simulink subsystem "RoboRio_Controls_sub"  (R2023b)
settings: Solver=VariableStepAuto  StartTime=0.0  StopTime=10.0  RelTol=1e-3
libraries: Autonomous_lib x1, simulink_extras x1, Disabled_lib x1, Teleop_lib x1, Test_lib x1
settings Model: Creator=USER  LastModifiedBy=FIRSTMentor

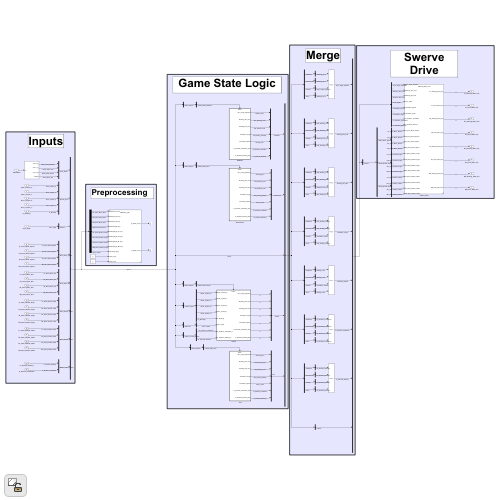
[thumbnail: Simulink's stored preview of the top-level diagram]
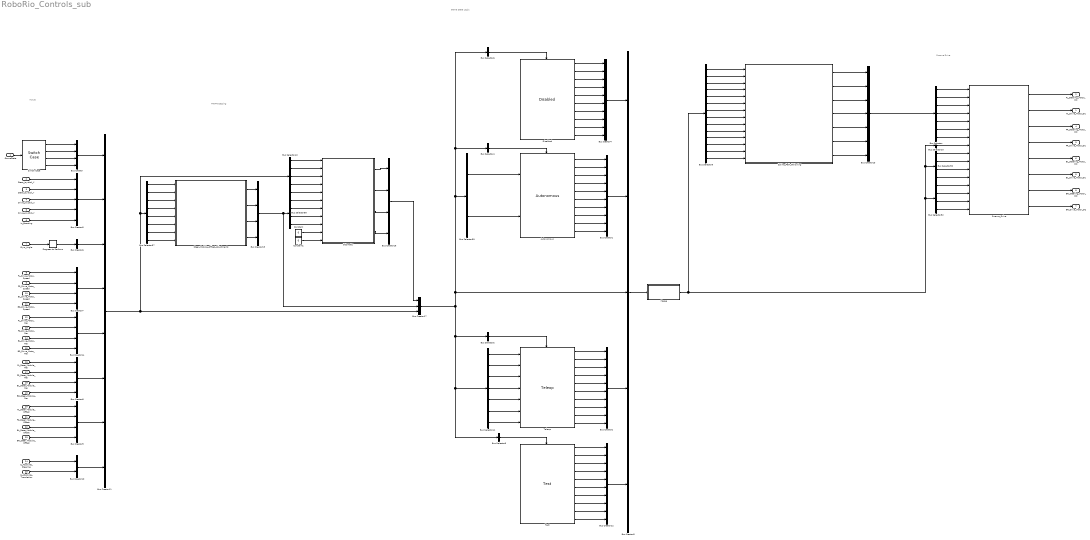
== system RoboRio_Controls_sub ==
  note: Game State Logic
  note: Swerve Drive
  note: Inputs
  note: Pre-Processing
  GameState : Inport
  Steer_Joystick_X : Inport  Port=2
  Steer_Joystick_Y : Inport  Port=3
  Drive_Joystick_X : Inport  Port=4
  Drive_Joystick_Y : Inport  Port=5
  Is_Boosting : Inport  Port=6
  Gyro_Angle : Inport  Port=7
  FL_Drive_Motor_Speed : Inport  Port=8
  FR_Drive_Motor_Speed : Inport  Port=9
  BL_Drive_Motor_Speed : Inport  Port=10
  BR_Drive_Motor_Speed : Inport  Port=11
  FL_Drive_Motor_Rev : Inport  Port=12
  FR_Drive_Motor_Rev : Inport  Port=13
  BL_Drive_Motor_Rev : Inport  Port=14
  BR_Drive_Motor_Rev : Inport  Port=15
  FL_Steer_Module_Rev : Inport  Port=16
  FR_Steer_Module_Rev : Inport  Port=17
  BL_Steer_Module_Rev : Inport  Port=18
  BR_Steer_Module_Rev : Inport  Port=19
  FL_Steer_Module_Offset : Inport  Port=20
  FR_Steer_Module_Offset : Inport  Port=21
  BL_Steer_Module_Offset : Inport  Port=22
  BR_Steer_Module_Offset : Inport  Port=23
  Is_Absolute_Steering : Inport  Port=24
  Is_Absolute_Translation : Inport  Port=25
  Autonomous : Autonomous_lib/Autonomous  SystemSampleTime=-1  VariantActivationTime=update diagram  AllowFlexibleInterface=on  Latency=0  AutoFrameSizeCalculation=off
  Bus Creator{,7..9,14..16} (7 alike) : BusCreator  Inputs=4
  Bus Creator{1..2,4,12} (4 alike) : BusCreator  Inputs=10
  Bus Creator10 : BusCreator  Inputs=2
  Bus Creator11 : BusCreator  Inputs=8
  Bus Creator13 : BusCreator  Inputs=7
  Bus Creator17 : BusCreator  Inputs=3
  Bus Creator3 : BusCreator  Inputs=5
  Bus Creator5 : BusCreator  Inputs=5
  Bus Creator6 : BusCreator  Inputs=1
  Bus Selector : BusSelector  OutputSignals=Steering_Abs_Cmd,Steering_Rel_Cmd,Translation_Speed,Translation_Angle,Is_Absolute_Translation,Is_Absolute_Steering,Gyro_Angle_Adjustment
  Bus Selector10 : BusSelector  OutputSignals=PreProcessing.Inputs.Sensors.Gyro_Angle
  Bus Selector2 : BusSelector  OutputSignals=Inputs.Game_States.Game_State_Teleop
  Bus Selector4 : BusSelector  OutputSignals=Inputs.Game_States.Game_State_Auto
  Bus Selector40 : BusSelector  OutputSignals=Sensors.Gyro_Angle,Drive_Motor_Revs.FL_Drive_Motor_Rev,Drive_Motor_Revs.FR_Drive_Motor_Rev,Drive_Motor_Revs.BL_Drive_Motor_Rev,Drive_Motor_Revs.BR_Drive_Motor_Rev
  Bus Selector41 : BusSelector  OutputSignals=Inputs.Human_Inputs.Steer_Joystick_X,Inputs.Human_Inputs.Steer_Joystick_Y,Inputs.Human_Inputs.Drive_Joystick_X,Inputs.Human_Inputs.Drive_Joystick_Y,Inputs.Human_Inputs.Is_Boosting,Inputs.Motion_Control_Modes.Is_Absolute_Translation,Inputs.Motion_Control_Modes.Is_Absolute_Steering
  Bus Selector50 : BusSelector  OutputSignals=PreProcessing.Inputs.Drive_Motor_Speeds.FL_Drive_Motor_Speed,PreProcessing.Inputs.Drive_Motor_Speeds.FR_Drive_Motor_Speed,PreProcessing.Inputs.Drive_Motor_Speeds.BL_Drive_Motor_Speed,PreProcessing.Inputs.Drive_Motor_Speeds.BR_Drive_Motor_Speed
  Bus Selector52 : BusSelector  OutputSignals=PreProcessing.Steer_Module_Angles.FL_Steer_Module_Angle,PreProcessing.Steer_Module_Angles.FR_Steer_Module_Angle,PreProcessing.Steer_Module_Angles.BL_Steer_Module_Angle,PreProcessing.Steer_Module_Angles.BR_Steer_Module_Angle
  Bus Selector57 : BusSelector  OutputSignals=Steer_Module_Revs.FL_Steer_Module_Rev,Steer_Module_Offsets.FL_Steer_Module_Offset,Steer_Module_Revs.FR_Steer_Module_Rev,Steer_Module_Offsets.FR_Steer_Module_Offset,Steer_Module_Revs.BL_Steer_Module_Rev,Steer_Module_Offsets.BL_Steer_Module_Offset,Steer_Module_Revs.BR_Steer_Module_Rev,Steer_Module_Offsets.BR_Steer_Module_Offset
  Bus Selector58 : BusSelector  OutputSignals=FL_Steer_Module_Angle,FR_Steer_Module_Angle,BL_Steer_Module_Angle,BR_Steer_Module_Angle
  Bus Selector59 : BusSelector  OutputSignals=Odometry.Odom_Position_X_global,Odometry.Odom_Position_Y_global
  Bus Selector6 : BusSelector  OutputSignals=Inputs.Game_States.Game_State_Disabled
  Bus Selector8 : BusSelector  OutputSignals=Inputs.Game_States.Game_State_Test
  Bus Selector9 : BusSelector  OutputSignals=Spline_Enable,Spline_Ref_Poses,Spline_Num_Poses,PreProcessing.Odometry.Odom_Position_X_global,PreProcessing.Odometry.Odom_Position_Y_global,PreProcessing.Odometry.Odom_Velocity_X_global,PreProcessing.Odometry.Odom_Velocity_Y_global,Steering_Abs_Cmd,Steering_Rel_Cmd,Translation_Speed,Translation_Angle,Is_Absolute_Translation,Is_Absolute_Steering,Gyro_Angle_Adjustment
  Constant : Constant  Value=0
  Constant1 : Constant  Value=0
  Degrees to Radians : simulink_extras/Transformations/Degrees to Radians
  Disabled : Disabled_lib/Disabled  SystemSampleTime=-1  VariantActivationTime=update diagram  AllowFlexibleInterface=on  Latency=0  AutoFrameSizeCalculation=off
  Merge : Subsystem
  Odometry : Subsystem  ReferencedSubsystem=Odometry_sub
  Spline_Path_Following : Subsystem  ReferencedSubsystem=Spline_Path_Following_sub
  Steer_Module_Offset_Adjustments : Subsystem  ReferencedSubsystem=Steer_Module_Offset_Adjustments_sub
  Swerve_Drive : Subsystem  ReferencedSubsystem=Swerve_Drive_sub
  Switch Case : SwitchCase  CaseConditions={0,1,2}
  Teleop : Teleop_lib/Teleop  SystemSampleTime=-1  VariantActivationTime=update diagram  AllowFlexibleInterface=on  Latency=0  AutoFrameSizeCalculation=off
  Test : Test_lib/Test  SystemSampleTime=-1  VariantActivationTime=update diagram  AllowFlexibleInterface=on  Latency=0  AutoFrameSizeCalculation=off
  FL_Drive_Motor_DC : Outport
  FL_Steering_Motor_DC : Outport  Port=2
  FR_Drive_Motor_DC : Outport  Port=3
  FR_Steering_Motor_DC : Outport  Port=4
  BL_Drive_Motor_DC : Outport  Port=5
  BL_Steering_Motor_DC : Outport  Port=6
  BR_Drive_Motor_DC : Outport  Port=7
  BR_Steering_Motor_DC : Outport  Port=8
  wires:
  Teleop/1 -> Bus Creator2/1
  Teleop/2 -> Bus Creator2/2
  Teleop/3 -> Bus Creator2/3
  Teleop/4 -> Bus Creator2/4
  Teleop/5 -> Bus Creator2/5
  Bus Creator4/1 -> Bus Creator3/1  "Disabled"
  Bus Creator1/1 -> Bus Creator3/2  "Autonomous"
  Bus Creator2/1 -> Bus Creator3/4  "Teleop"
  Switch Case/1 -> Bus Creator/1  "Game_State_Disabled"
  Switch Case/2 -> Bus Creator/2  "Game_State_Auto"
  Switch Case/3 -> Bus Creator/3  "Game_State_Teleop"
  GameState/1 -> Switch Case/1
  Bus Creator12/1 -> Bus Creator3/5  "Test"
  Switch Case/4 -> Bus Creator/4  "Game_State_Test"
  Steer_Joystick_Y/1 -> Bus Creator5/2  "Steer_Joystick_Y"
  Steer_Joystick_X/1 -> Bus Creator5/1  "Steer_Joystick_X"
  Drive_Joystick_X/1 -> Bus Creator5/3  "Drive_Joystick_X"
  Drive_Joystick_Y/1 -> Bus Creator5/4  "Drive_Joystick_Y"
  Gyro_Angle/1 -> Degrees to Radians/1
  Bus Creator5/1 -> Bus Creator11/2  "Human_Inputs"
  Bus Creator6/1 -> Bus Creator11/3  "Sensors"
  FL_Drive_Motor_Speed/1 -> Bus Creator7/1  "FL_Drive_Motor_Speed"
  FR_Drive_Motor_Speed/1 -> Bus Creator7/2  "FR_Drive_Motor_Speed"
  BL_Drive_Motor_Speed/1 -> Bus Creator7/3  "BL_Drive_Motor_Speed"
  BR_Drive_Motor_Speed/1 -> Bus Creator7/4  "BR_Drive_Motor_Speed"
  FL_Steer_Module_Rev/1 -> Bus Creator8/1  "FL_Steer_Module_Rev"
  BL_Steer_Module_Rev/1 -> Bus Creator8/3  "BL_Steer_Module_Rev"
  BR_Steer_Module_Rev/1 -> Bus Creator8/4  "BR_Steer_Module_Rev"
  FR_Steer_Module_Rev/1 -> Bus Creator8/2  "FR_Steer_Module_Rev"
  Bus Creator7/1 -> Bus Creator11/4  "Drive_Motor_Speeds"
  Bus Creator8/1 -> Bus Creator11/6  "Steer_Module_Revs"
  FL_Steer_Module_Offset/1 -> Bus Creator9/1  "FL_Steer_Module_Offset"
  FR_Steer_Module_Offset/1 -> Bus Creator9/2  "FR_Steer_Module_Offset"
  BL_Steer_Module_Offset/1 -> Bus Creator9/3  "BL_Steer_Module_Offset"
  BR_Steer_Module_Offset/1 -> Bus Creator9/4  "BR_Steer_Module_Offset"
  Bus Creator9/1 -> Bus Creator11/7  "Steer_Module_Offsets"
  Is_Absolute_Steering/1 -> Bus Creator10/1  "Is_Absolute_Steering"
  Is_Absolute_Translation/1 -> Bus Creator10/2  "Is_Absolute_Translation"
  Bus Creator10/1 -> Bus Creator11/8  "Motion_Control_Modes"
  Bus Selector41/1 -> Teleop/1  "<Steer_Joystick_X>"
  Bus Selector41/2 -> Teleop/2  "<Steer_Joystick_Y>"
  Bus Selector41/3 -> Teleop/3  "<Drive_Joystick_X>"
  Bus Selector41/4 -> Teleop/4  "<Drive_Joystick_Y>"
  Teleop/6 -> Bus Creator2/6
  Teleop/7 -> Bus Creator2/7
  Autonomous/2 -> Bus Creator1/2
  Autonomous/4 -> Bus Creator1/4
  Autonomous/1 -> Bus Creator1/1
  Autonomous/5 -> Bus Creator1/5
  Autonomous/7 -> Bus Creator1/7
  Autonomous/3 -> Bus Creator1/3
  Autonomous/6 -> Bus Creator1/6
  Disabled/2 -> Bus Creator4/2
  Disabled/4 -> Bus Creator4/4
  Disabled/1 -> Bus Creator4/1
  Disabled/5 -> Bus Creator4/5
  Disabled/7 -> Bus Creator4/7
  Disabled/3 -> Bus Creator4/3
  Disabled/6 -> Bus Creator4/6
  Test/2 -> Bus Creator12/2
  Test/4 -> Bus Creator12/4
  Test/1 -> Bus Creator12/1
  Test/5 -> Bus Creator12/5
  Test/7 -> Bus Creator12/7
  Test/3 -> Bus Creator12/3
  Test/6 -> Bus Creator12/6
  Bus Creator/1 -> Bus Creator11/1  "Game_States"
  Bus Selector2/1 -> Teleop/Action  "<Game_State_Teleop>"
  Bus Selector4/1 -> Autonomous/Action  "<Game_State_Auto>"
  Bus Selector6/1 -> Disabled/Action  "<Game_State_Disabled>"
  Bus Selector8/1 -> Test/Action  "<Game_State_Test>"
  Bus Selector50/4 -> Swerve_Drive/12  "<BR_Drive_Motor_Speed>"
  Bus Selector50/3 -> Swerve_Drive/11  "<BL_Drive_Motor_Speed>"
  Bus Selector50/2 -> Swerve_Drive/10  "<FR_Drive_Motor_Speed>"
  Bus Selector50/1 -> Swerve_Drive/9  "<FL_Drive_Motor_Speed>"
  Swerve_Drive/1 -> FL_Steering_Motor_DC/1
  Swerve_Drive/2 -> FL_Drive_Motor_DC/1
  Swerve_Drive/3 -> FR_Steering_Motor_DC/1
  Swerve_Drive/4 -> FR_Drive_Motor_DC/1
  Swerve_Drive/5 -> BL_Steering_Motor_DC/1
  Swerve_Drive/6 -> BL_Drive_Motor_DC/1
  Swerve_Drive/7 -> BR_Steering_Motor_DC/1
  Swerve_Drive/8 -> BR_Drive_Motor_DC/1
  Is_Boosting/1 -> Bus Creator5/5  "Is_Boosting"
  Bus Selector41/5 -> Teleop/5  "<Is_Boosting>"
  Bus Creator14/1 -> Bus Creator11/5  "Drive_Motor_Revs"
  FL_Drive_Motor_Rev/1 -> Bus Creator14/1  "FL_Drive_Motor_Rev"
  FR_Drive_Motor_Rev/1 -> Bus Creator14/2  "FR_Drive_Motor_Rev"
  BL_Drive_Motor_Rev/1 -> Bus Creator14/3  "BL_Drive_Motor_Rev"
  BR_Drive_Motor_Rev/1 -> Bus Creator14/4  "BR_Drive_Motor_Rev"
  Bus Selector40/2 -> Odometry/2  "<FL_Drive_Motor_Rev>"
  Bus Selector40/3 -> Odometry/3  "<FR_Drive_Motor_Rev>"
  Bus Selector40/4 -> Odometry/4  "<BL_Drive_Motor_Rev>"
  Bus Selector40/5 -> Odometry/5  "<BR_Drive_Motor_Rev>"
  Bus Selector40/1 -> Odometry/1  "<Gyro_Angle>"
  Constant1/1 -> Odometry/11
  Constant/1 -> Odometry/10
  Bus Selector57/1 -> Steer_Module_Offset_Adjustments/1  "<FL_Steer_Module_Rev>"
  Bus Selector57/2 -> Steer_Module_Offset_Adjustments/2  "<FL_Steer_Module_Offset>"
  Bus Selector57/3 -> Steer_Module_Offset_Adjustments/3  "<FR_Steer_Module_Rev>"
  Bus Selector57/4 -> Steer_Module_Offset_Adjustments/4  "<FR_Steer_Module_Offset>"
  Bus Selector57/5 -> Steer_Module_Offset_Adjustments/5  "<BL_Steer_Module_Rev>"
  Bus Selector57/6 -> Steer_Module_Offset_Adjustments/6  "<BL_Steer_Module_Offset>"
  Bus Selector57/7 -> Steer_Module_Offset_Adjustments/7  "<BR_Steer_Module_Rev>"
  Bus Selector57/8 -> Steer_Module_Offset_Adjustments/8  "<BR_Steer_Module_Offset>"
  Steer_Module_Offset_Adjustments/2 -> Bus Creator15/2
  Steer_Module_Offset_Adjustments/1 -> Bus Creator15/1
  Steer_Module_Offset_Adjustments/3 -> Bus Creator15/3
  Steer_Module_Offset_Adjustments/4 -> Bus Creator15/4
  Bus Creator15/1 -> Bus Selector58/1, Bus Creator17/2  "Steer_Module_Angles"
  Bus Selector58/1 -> Odometry/6  "<FL_Steer_Module_Angle>"
  Bus Selector58/2 -> Odometry/7  "<FR_Steer_Module_Angle>"
  Bus Selector58/3 -> Odometry/8  "<BL_Steer_Module_Angle>"
  Bus Selector58/4 -> Odometry/9  "<BR_Steer_Module_Angle>"
  Odometry/1 -> Bus Creator16/1
  Odometry/2 -> Bus Creator16/2
  Bus Creator16/1 -> Bus Creator17/1  "Odometry"
  Bus Creator11/1 -> Bus Creator17/3, Bus Selector57/1, Bus Selector40/1  "Inputs"
  Bus Selector52/1 -> Swerve_Drive/13  "<FL_Steer_Module_Angle>"
  Bus Selector52/2 -> Swerve_Drive/14  "<FR_Steer_Module_Angle>"
  Bus Selector52/3 -> Swerve_Drive/15  "<BL_Steer_Module_Angle>"
  Bus Selector52/4 -> Swerve_Drive/16  "<BR_Steer_Module_Angle>"
  Degrees to Radians/1 -> Bus Creator6/1  "Gyro_Angle"
  Bus Creator17/1 -> Bus Selector8/1, Bus Selector41/1, Bus Selector2/1, Bus Creator3/3, Bus Selector59/1, Bus Selector4/1, Bus Selector6/1  "PreProcessing"
  Disabled/8 -> Bus Creator4/8
  Disabled/9 -> Bus Creator4/9
  Disabled/10 -> Bus Creator4/10
  Autonomous/8 -> Bus Creator1/8
  Autonomous/9 -> Bus Creator1/9
  Autonomous/10 -> Bus Creator1/10
  Teleop/8 -> Bus Creator2/8
  Teleop/9 -> Bus Creator2/9
  Teleop/10 -> Bus Creator2/10
  Test/8 -> Bus Creator12/8
  Test/9 -> Bus Creator12/9
  Test/10 -> Bus Creator12/10
  Merge/1(Bus_Out) -> Bus Selector52/1, Bus Selector50/1, Bus Selector10/1, Bus Selector9/1
  Bus Creator3/1 -> Merge/1(Bus_In)
  Odometry/3 -> Bus Creator16/3
  Odometry/4 -> Bus Creator16/4
  Bus Selector10/1 -> Swerve_Drive/8  "<Gyro_Angle>"
  Bus Selector59/1 -> Autonomous/1  "<Odom_Position_X_global>"
  Bus Selector59/2 -> Autonomous/2  "<Odom_Position_Y_global>"
  Bus Selector41/7 -> Teleop/7  "<Is_Absolute_Steering>"
  Bus Selector41/6 -> Teleop/6  "<Is_Absolute_Translation>"
  Bus Selector9/1 -> Spline_Path_Following/1  "<Spline_Enable>"
  Bus Selector9/2 -> Spline_Path_Following/2  "<Spline_Ref_Poses>"
  Bus Selector9/3 -> Spline_Path_Following/3  "<Spline_Num_Poses>"
  Bus Selector9/4 -> Spline_Path_Following/4  "<Odom_Position_X_global>"
  Bus Selector9/5 -> Spline_Path_Following/5  "<Odom_Position_Y_global>"
  Bus Selector9/6 -> Spline_Path_Following/6  "<Odom_Velocity_X_global>"
  Bus Selector9/7 -> Spline_Path_Following/7  "<Odom_Velocity_Y_global>"
  Bus Selector9/8 -> Spline_Path_Following/8  "<Steering_Abs_Cmd>"
  Bus Selector9/9 -> Spline_Path_Following/9  "<Steering_Rel_Cmd>"
  Bus Selector9/10 -> Spline_Path_Following/10  "<Translation_Speed>"
  Bus Selector9/11 -> Spline_Path_Following/11  "<Translation_Angle>"
  Bus Selector9/12 -> Spline_Path_Following/12  "<Is_Absolute_Translation>"
  Bus Selector9/13 -> Spline_Path_Following/13  "<Is_Absolute_Steering>"
  Bus Selector9/14 -> Spline_Path_Following/14  "<Gyro_Angle_Adjustment>"
  Spline_Path_Following/1 -> Bus Creator13/1
  Spline_Path_Following/2 -> Bus Creator13/2
  Spline_Path_Following/3 -> Bus Creator13/3
  Spline_Path_Following/4 -> Bus Creator13/4
  Spline_Path_Following/5 -> Bus Creator13/5
  Spline_Path_Following/6 -> Bus Creator13/6
  Spline_Path_Following/7 -> Bus Creator13/7
  Bus Creator13/1 -> Bus Selector/1
  Bus Selector/5 -> Swerve_Drive/5  "<Is_Absolute_Translation>"
  Bus Selector/4 -> Swerve_Drive/4  "<Translation_Angle>"
  Bus Selector/6 -> Swerve_Drive/6  "<Is_Absolute_Steering>"
  Bus Selector/3 -> Swerve_Drive/3  "<Translation_Speed>"
  Bus Selector/7 -> Swerve_Drive/7  "<Gyro_Angle_Adjustment>"
  Bus Selector/2 -> Swerve_Drive/2  "<Steering_Rel_Cmd>"
  Bus Selector/1 -> Swerve_Drive/1  "<Steering_Abs_Cmd>"

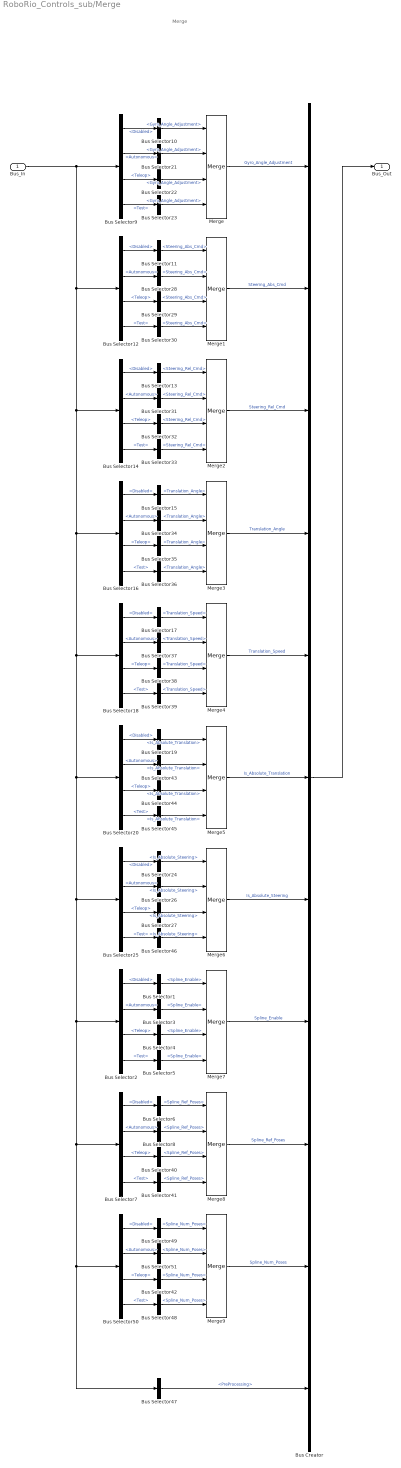
== system RoboRio_Controls_sub/Merge ==
  note: Merge
  Bus_In : Inport
  Bus Creator : BusCreator  Inputs=11
  Bus Selector{1,3..5} (4 alike) : BusSelector  OutputSignals=Spline_Enable
  Bus Selector{10,21..23} (4 alike) : BusSelector  OutputSignals=Gyro_Angle_Adjustment
  Bus Selector{11,28..30} (4 alike) : BusSelector  OutputSignals=Steering_Abs_Cmd
  Bus Selector{2,7,9,12,14,16,18,20,25,50} (10 alike) : BusSelector  OutputSignals=Disabled,Autonomous,Teleop,Test
  Bus Selector{13,31..33} (4 alike) : BusSelector  OutputSignals=Steering_Rel_Cmd
  Bus Selector{15,34..36} (4 alike) : BusSelector  OutputSignals=Translation_Angle
  Bus Selector{17,37..39} (4 alike) : BusSelector  OutputSignals=Translation_Speed
  Bus Selector{19,43..45} (4 alike) : BusSelector  OutputSignals=Is_Absolute_Translation
  Bus Selector{24,26..27,46} (4 alike) : BusSelector  OutputSignals=Is_Absolute_Steering
  Bus Selector{6,8,40..41} (4 alike) : BusSelector  OutputSignals=Spline_Ref_Poses
  Bus Selector{42,48..49,51} (4 alike) : BusSelector  OutputSignals=Spline_Num_Poses
  Bus Selector47 : BusSelector  OutputSignals=PreProcessing
  Merge{,1..9} (10 alike) : Merge  Inputs=4
  Bus_Out : Outport
  wires:
  Merge9/1 -> Bus Creator/10  "Spline_Num_Poses"
  Bus Selector48/1 -> Merge9/4  "<Spline_Num_Poses>"
  Bus Selector50/1 -> Bus Selector49/1  "<Disabled>"
  Bus Selector42/1 -> Merge9/3  "<Spline_Num_Poses>"
  Bus Selector49/1 -> Merge9/1  "<Spline_Num_Poses>"
  Bus Selector51/1 -> Merge9/2  "<Spline_Num_Poses>"
  Bus Selector50/4 -> Bus Selector48/1  "<Test>"
  Bus Selector50/3 -> Bus Selector42/1  "<Teleop>"
  Bus Selector50/2 -> Bus Selector51/1  "<Autonomous>"
  Merge8/1 -> Bus Creator/9  "Spline_Ref_Poses"
  Bus Selector7/2 -> Bus Selector8/1  "<Autonomous>"
  Bus Selector7/3 -> Bus Selector40/1  "<Teleop>"
  Bus Selector7/4 -> Bus Selector41/1  "<Test>"
  Bus Selector8/1 -> Merge8/2  "<Spline_Ref_Poses>"
  Bus Selector6/1 -> Merge8/1  "<Spline_Ref_Poses>"
  Bus Selector40/1 -> Merge8/3  "<Spline_Ref_Poses>"
  Bus Selector7/1 -> Bus Selector6/1  "<Disabled>"
  Bus Selector41/1 -> Merge8/4  "<Spline_Ref_Poses>"
  Merge7/1 -> Bus Creator/8  "Spline_Enable"
  Bus Selector5/1 -> Merge7/4  "<Spline_Enable>"
  Bus Selector2/1 -> Bus Selector1/1  "<Disabled>"
  Bus Selector4/1 -> Merge7/3  "<Spline_Enable>"
  Bus Selector1/1 -> Merge7/1  "<Spline_Enable>"
  Bus Selector3/1 -> Merge7/2  "<Spline_Enable>"
  Bus Selector2/4 -> Bus Selector5/1  "<Test>"
  Bus Selector2/3 -> Bus Selector4/1  "<Teleop>"
  Bus Selector2/2 -> Bus Selector3/1  "<Autonomous>"
  Bus Creator/1 -> Bus_Out/1
  Bus Selector29/1 -> Merge1/3  "<Steering_Abs_Cmd>"
  Bus Selector25/2 -> Bus Selector26/1  "<Autonomous>"
  Bus Selector25/3 -> Bus Selector27/1  "<Teleop>"
  Bus Selector14/3 -> Bus Selector32/1  "<Teleop>"
  Bus Selector16/3 -> Bus Selector35/1  "<Teleop>"
  Bus Selector16/4 -> Bus Selector36/1  "<Test>"
  Bus Selector20/1 -> Bus Selector19/1  "<Disabled>"
  Merge1/1 -> Bus Creator/2  "Steering_Abs_Cmd"
  Bus Selector34/1 -> Merge3/2  "<Translation_Angle>"
  Merge/1 -> Bus Creator/1  "Gyro_Angle_Adjustment"
  Bus Selector17/1 -> Merge4/1  "<Translation_Speed>"
  Bus Selector15/1 -> Merge3/1  "<Translation_Angle>"
  Bus Selector21/1 -> Merge/2  "<Gyro_Angle_Adjustment>"
  Bus Selector9/3 -> Bus Selector22/1  "<Teleop>"
  Bus Selector20/2 -> Bus Selector43/1  "<Autonomous>"
  Bus Selector14/1 -> Bus Selector13/1  "<Disabled>"
  Bus Selector23/1 -> Merge/4  "<Gyro_Angle_Adjustment>"
  Bus Selector20/4 -> Bus Selector45/1  "<Test>"
  Bus Selector10/1 -> Merge/1  "<Gyro_Angle_Adjustment>"
  Merge5/1 -> Bus Creator/6  "Is_Absolute_Translation"
  Bus Selector36/1 -> Merge3/4  "<Translation_Angle>"
  Bus Selector47/1 -> Bus Creator/11  "<PreProcessing>"
  Bus Selector12/1 -> Bus Selector11/1  "<Disabled>"
  Bus Selector16/2 -> Bus Selector34/1  "<Autonomous>"
  Bus Selector22/1 -> Merge/3  "<Gyro_Angle_Adjustment>"
  Bus Selector37/1 -> Merge4/2  "<Translation_Speed>"
  Bus Selector25/4 -> Bus Selector46/1  "<Test>"
  Bus Selector18/3 -> Bus Selector38/1  "<Teleop>"
  Bus Selector20/3 -> Bus Selector44/1  "<Teleop>"
  Bus Selector39/1 -> Merge4/4  "<Translation_Speed>"
  Bus Selector16/1 -> Bus Selector15/1  "<Disabled>"
  Bus Selector13/1 -> Merge2/1  "<Steering_Rel_Cmd>"
  Bus Selector30/1 -> Merge1/4  "<Steering_Abs_Cmd>"
  Bus Selector26/1 -> Merge6/2  "<Is_Absolute_Steering>"
  Merge6/1 -> Bus Creator/7  "Is_Absolute_Steering"
  Bus Selector18/1 -> Bus Selector17/1  "<Disabled>"
  Bus Selector45/1 -> Merge5/4  "<Is_Absolute_Translation>"
  Bus Selector12/3 -> Bus Selector29/1  "<Teleop>"
  Bus Selector18/2 -> Bus Selector37/1  "<Autonomous>"
  Bus Selector43/1 -> Merge5/2  "<Is_Absolute_Translation>"
  Bus Selector19/1 -> Merge5/1  "<Is_Absolute_Translation>"
  Bus Selector35/1 -> Merge3/3  "<Translation_Angle>"
  Merge3/1 -> Bus Creator/4  "Translation_Angle"
  Bus Selector28/1 -> Merge1/2  "<Steering_Abs_Cmd>"
  Bus Selector14/2 -> Bus Selector31/1  "<Autonomous>"
  Bus Selector32/1 -> Merge2/3  "<Steering_Rel_Cmd>"
  Merge4/1 -> Bus Creator/5  "Translation_Speed"
  Bus Selector12/2 -> Bus Selector28/1  "<Autonomous>"
  Bus Selector14/4 -> Bus Selector33/1  "<Test>"
  Bus Selector44/1 -> Merge5/3  "<Is_Absolute_Translation>"
  Bus Selector24/1 -> Merge6/1  "<Is_Absolute_Steering>"
  Bus Selector11/1 -> Merge1/1  "<Steering_Abs_Cmd>"
  Bus Selector9/2 -> Bus Selector21/1  "<Autonomous>"
  Bus Selector31/1 -> Merge2/2  "<Steering_Rel_Cmd>"
  Bus Selector27/1 -> Merge6/3  "<Is_Absolute_Steering>"
  Bus Selector25/1 -> Bus Selector24/1  "<Disabled>"
  Bus Selector18/4 -> Bus Selector39/1  "<Test>"
  Bus Selector46/1 -> Merge6/4  "<Is_Absolute_Steering>"
  Bus Selector9/4 -> Bus Selector23/1  "<Test>"
  Bus Selector38/1 -> Merge4/3  "<Translation_Speed>"
  Bus Selector33/1 -> Merge2/4  "<Steering_Rel_Cmd>"
  Bus Selector9/1 -> Bus Selector10/1  "<Disabled>"
  Bus_In/1 -> Bus Selector9/1, Bus Selector12/1, Bus Selector14/1, Bus Selector16/1, Bus Selector18/1, Bus Selector20/1, Bus Selector25/1, Bus Selector47/1, Bus Selector50/1, Bus Selector7/1, Bus Selector2/1
  Bus Selector12/4 -> Bus Selector30/1  "<Test>"
  Merge2/1 -> Bus Creator/3  "Steering_Rel_Cmd"
